simulink model "ISS_single"  (R2015b)
settings: Solver=VariableStepAuto  StartTime=0.0  StopTime=50  RelTol=1e-3
values from neighbouring files (symbols this model uses):
  bHI = 0    [Initiation.m]
  bWall = block.DialogPrm(2).Data    [HapticController.m]    (also in Initiation.m = 0; VirtualEnvironment5.m)
  dof = block.DialogPrm(2).Data    [Controller.m]    (also in Controller1.m; Controller_more.m = block.DialogPrm(3).Data; Initiation.m = 1; Parameters.m = 1)
  kWall = block.DialogPrm(1).Data    [HapticController.m]    (also in Initiation.m = 5000; VirtualEnvironment5.m)
  m = 1    [Initiation.m]
  nWall = block.DialogPrm(6).Data    [Controller1.m]    (also in HapticController.m = block.DialogPrm(3).Data; Initial_Conditions.m = -1; Initiation.m = -1; MoreConservative.m = block.DialogPrm(5).Data)
  tau = 0.003    [Initiation.m]    (also in controller.m = block.DialogPrm(1).Data)
  tsampling = block.DialogPrm(3).Data    [Controller.m]    (also in Controller1.m; Controller_more.m = block.DialogPrm(4).Data; HapticController.m = block.DialogPrm(6).Data; Initial_Conditions.m = 0.001)
  x0 = block.DialogPrm(5).Data    [HapticDevice.m]    (also in HumanOperator.m; LessConservative.m = block.DialogPrm(3).Data; MoreConservative.m = block.DialogPrm(3).Data)
  xWall = 0.126    [Initiation.m]    (also in MoreConservative.m = block.DialogPrm(4).Data; Parameters.m = [1 2 3 4 5 6 7 8]*0.0005; VirtualEnvironment.m = block.DialogPrm(3).Data; VirtualEnvironment5.m = block.DialogPrm(4).Data)
undefined symbols (not defined in the file or in its folder): x_dot0
settings Model: Creator=TOSHIBA  LastModifiedBy=TOSHIBA

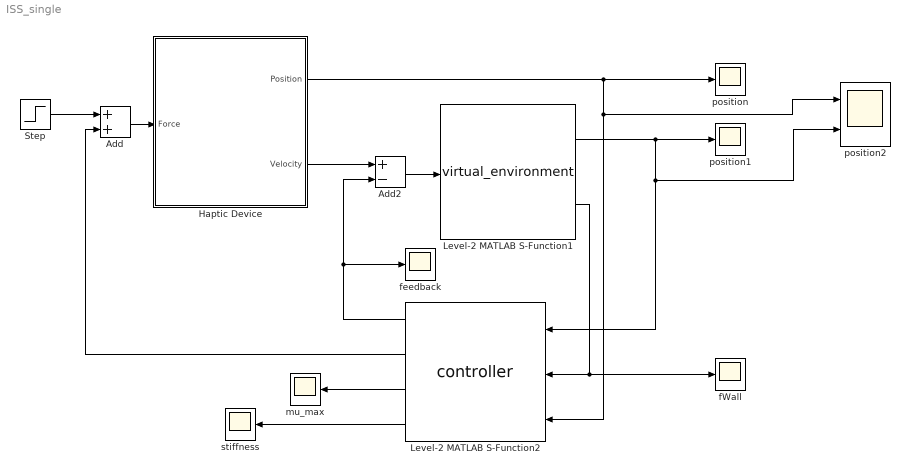
== system ISS_single ==
  Add : Sum
  Add2 : Sum  Inputs=+-
  Haptic Device : Subsystem
  Level-2 MATLAB S-Function1 : M-S-Function  FunctionName=virtual_environment  Parameters=kWall,bWall,nWall,xWall,x_dot0,x0,dof,tsampling
  Level-2 MATLAB S-Function2 : M-S-Function  FunctionName=controller  Parameters=tau,dof,tsampling,x0,xWall,nWall
  Step : Step  Time=0.35  After=-10  SampleTime=0
  fWall : Scope
  feedback : Scope
  mu_max : Scope
  position : Scope
  position1 : Scope
  position2 : Scope  NumInputPorts=2
  stiffness : Scope
  wires:
  Level-2 MATLAB S-Function1/1 -> position2/2, Level-2 MATLAB S-Function2/1, position1/1
  Step/1 -> Add/1
  Add/1 -> Haptic Device/1(Force)
  Level-2 MATLAB S-Function1/2 -> fWall/1, Level-2 MATLAB S-Function2/2
  Level-2 MATLAB S-Function2/2 -> Add/2
  Add2/1 -> Level-2 MATLAB S-Function1/1
  Level-2 MATLAB S-Function2/3 -> mu_max/1
  Level-2 MATLAB S-Function2/1 -> Add2/2, feedback/1
  Haptic Device/2(Velocity) -> Add2/1
  Haptic Device/1(Position) -> position2/1, Level-2 MATLAB S-Function2/3, position/1
  Level-2 MATLAB S-Function2/4 -> stiffness/1

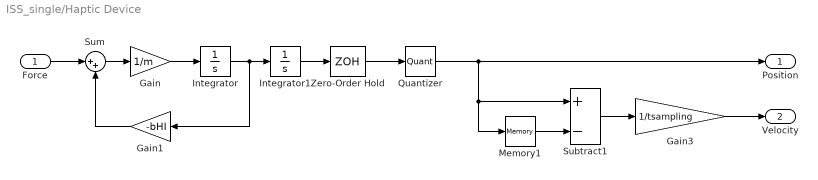
== system ISS_single/Haptic Device ==
  Force : Inport
  Gain : Gain  Gain=1/m
  Gain1 : Gain  Gain=-bHI
  Gain3 : Gain  Gain=1/tsampling
  Integrator : Integrator  InitialCondition=x_dot0
  Integrator1 : Integrator  InitialCondition=x0
  Memory1 : Memory  X0=x0
  Quantizer : Quantizer  QuantizationInterval=0.00005
  Subtract1 : Sum  Inputs=+-
  Sum : Sum  Inputs=|++
  Zero-Order Hold : ZeroOrderHold  SampleTime=tsampling
  Position : Outport
  Velocity : Outport  Port=2
  wires:
  Integrator1/1 -> Zero-Order Hold/1
  Gain/1 -> Integrator/1
  Sum/1 -> Gain/1
  Gain1/1 -> Sum/2
  Integrator/1 -> Gain1/1, Integrator1/1
  Force/1 -> Sum/1
  Subtract1/1 -> Gain3/1
  Memory1/1 -> Subtract1/2
  Gain3/1 -> Velocity/1
  Zero-Order Hold/1 -> Quantizer/1
  Quantizer/1 -> Memory1/1, Subtract1/1, Position/1
